simulink model "para_id_0_mod_corriente"  (R2018a)
settings: Solver=VariableStepAuto  StartTime=0.0  StopTime=10.0  RelTol=1e-3
values from neighbouring files (symbols this model uses):
  Beq = bm+(bl)/r^2    (= 1.5e-05)    [c4ModeloCompleto_var.m]
  Cts = .818    (= 0.818)    [c4ModeloCompleto.m]    (also in c4ModeloCompleto_var.m)
  Jeq = Jm+(Jl/r^2)    (= 5.65099476805e-06)    [c4ModeloCompleto_var.m]
  Ld = 6.6    [c4ModeloCompleto.m]    (also in c4ModeloCompleto_var.m = 0.0066)
  Lq = 5.8    [c4ModeloCompleto.m]    (also in c4ModeloCompleto_var.m = 0.0058)
  Pp = 3    [c4ModeloCompleto.m]    (also in c4ModeloCompleto_var.m)
  r = 314.3008    [c4ModeloCompleto.m]    (also in c4ModeloCompleto_var.m)
  Rs = 1.02    [c4ModeloCompleto_var.m]
  Rts_amb = 146.7    [c4ModeloCompleto.m]    (also in c4ModeloCompleto_var.m)
undefined symbols (not defined in the file or in its folder): L0
settings Model: Creator=agustin  LastModifiedBy=emanuel
settings CodeAppCC: StateflowObjectComments=on

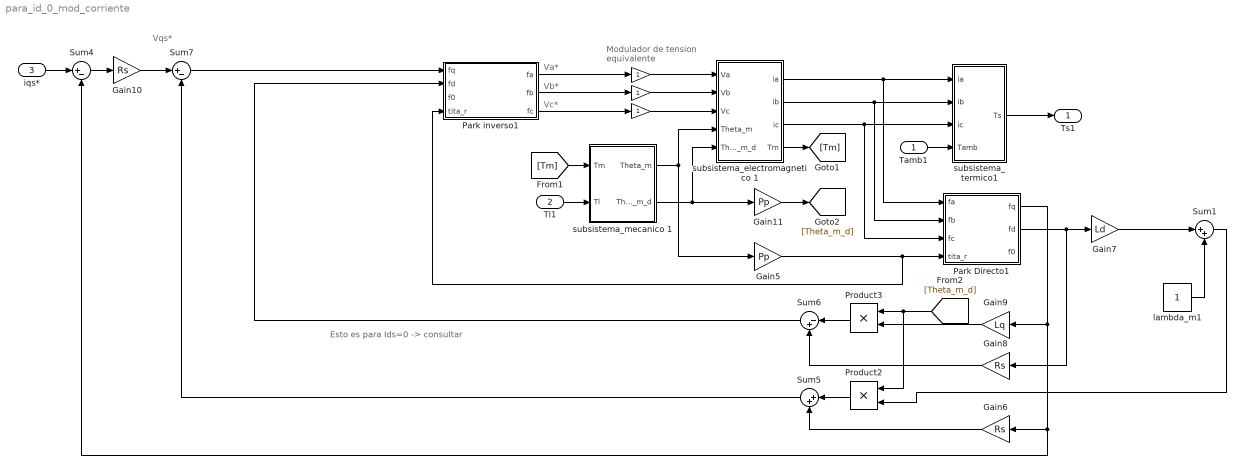
== system para_id_0_mod_corriente ==
  note: Vqs*
  note: Modulador de tension
      | equivalente
  note: Vc*
  note: Vb*
  note: Va*
  note: Esto es para Ids=0 -> consultar
  Tamb1 : Inport
  Tl1 : Inport  Port=2
  iqs* : Inport  Port=3
  " " : Gain
  " " : Gain
  " " : Gain
  Gain10 : Gain  Gain=Rs
  Gain11 : Gain  Gain=Pp
  Gain5 : Gain  Gain=Pp
  Gain6 : Gain  Gain=Rs
  Gain7 : Gain  Gain=Ld
  Gain8 : Gain  Gain=Rs
  Gain9 : Gain  Gain=Lq
  Park Directo1 : MATLAB Function  TreatAsAtomicUnit=on
  Park inverso1 : MATLAB Function  TreatAsAtomicUnit=on
  Product2 : Product
  Product3 : Product
  Sum1 : Sum  Inputs=|++
  Sum4 : Sum  Inputs=|+-
  Sum5 : Sum  Inputs=|++
  Sum6 : Sum  Inputs=|-+
  Sum7 : Sum  Inputs=|+-
  lambda_m1 : Constant
  subsistema_electromagnetico 1 : Subsystem
  subsistema_mecanico 1 : Subsystem
  subsistema_termico1 : Subsystem
  Ts1 : Outport
  wires:
  subsistema_mecanico 1/2("Theta_m_d ") -> Gain11/1, subsistema_electromagnetico 1/5(Theta_m_d)
  subsistema_termico1/1(Ts) -> Ts1/1
  Tamb1/1 -> subsistema_termico1/4(Tamb)
  subsistema_mecanico 1/1("Theta_m ") -> Gain5/1, subsistema_electromagnetico 1/4(Theta_m)
  Park inverso1/1(fa) -> " "/1
  Park inverso1/2(fb) -> " "/1
  Park inverso1/3(fc) -> " "/1
  subsistema_electromagnetico 1/1(ia) -> subsistema_termico1/1(ia), Park Directo1/1(fa)
  subsistema_electromagnetico 1/2(ib) -> Park Directo1/2(fb), subsistema_termico1/2(ib)
  subsistema_electromagnetico 1/3(ic) -> Park Directo1/3(fc), subsistema_termico1/3("ic ")
  Gain5/1 -> Park inverso1/4(tita_r), Park Directo1/4(tita_r)
  [Tm] -> subsistema_mecanico 1/1(Tm)
  subsistema_electromagnetico 1/4(Tm) -> [Tm]
  Tl1/1 -> subsistema_mecanico 1/2(Tl)
  Park Directo1/1(fq) -> Gain9/1, Sum4/2, Gain6/1
  Park Directo1/2(fd) -> Gain8/1, Gain7/1
  Gain7/1 -> Sum1/1
  lambda_m1/1 -> Sum1/2
  Sum1/1 -> Product2/2
  Gain6/1 -> Sum5/2
  Product2/1 -> Sum5/1
  Sum5/1 -> Sum7/2
  Gain8/1 -> Sum6/2
  Gain9/1 -> Product3/2
  Product3/1 -> Sum6/1
  Sum6/1 -> Park inverso1/2(fd)
  " "/1 -> subsistema_electromagnetico 1/1(Va)
  " "/1 -> subsistema_electromagnetico 1/3(Vc)
  " "/1 -> subsistema_electromagnetico 1/2(Vb)
  iqs*/1 -> Sum4/1
  Sum4/1 -> Gain10/1
  Gain10/1 -> Sum7/1
  [Theta_m_d] -> Product2/1, Product3/1
  Gain11/1 -> [Theta_m_d]
  Sum7/1 -> Park inverso1/1(fq)

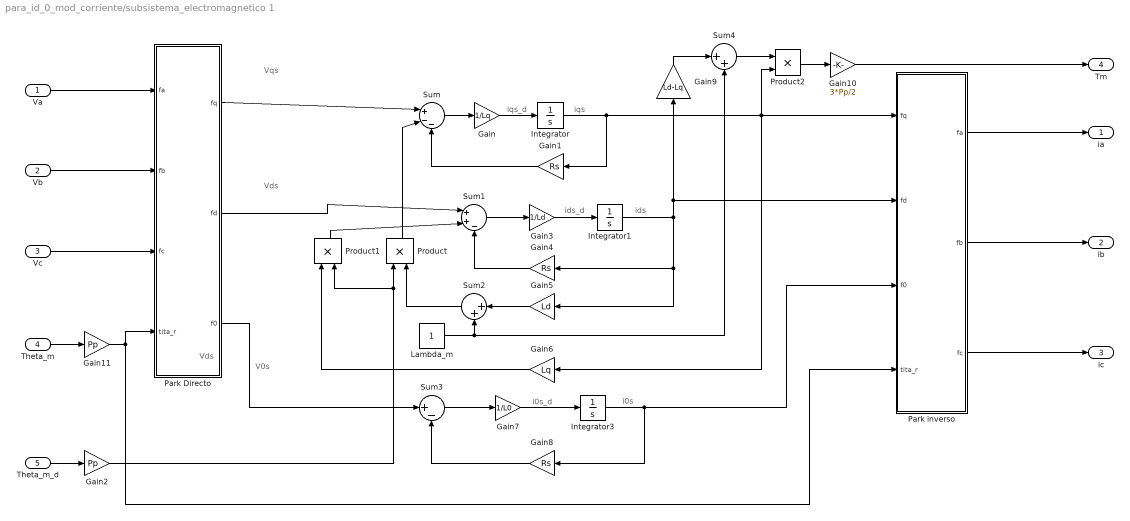
== system para_id_0_mod_corriente/subsistema_electromagnetico 1 ==
  note: Vds
  note: Vqs
  note: V0s
  note: Vds
  note: i0s
  note: i0s_d
  note: ids_d
  note: ids
  note: iqs
  note: iqs_d
  Va : Inport
  Vb : Inport  Port=2
  Vc : Inport  Port=3
  Theta_m : Inport  Port=4
  Theta_m_d : Inport  Port=5
  Gain : Gain  Gain=1/Lq
  Gain1 : Gain  Gain=Rs
  Gain10 : Gain  Gain=3*Pp/2
  Gain11 : Gain  Gain=Pp
  Gain2 : Gain  Gain=Pp
  Gain3 : Gain  Gain=1/Ld
  Gain4 : Gain  Gain=Rs
  Gain5 : Gain  Gain=Ld
  Gain6 : Gain  Gain=Lq
  Gain7 : Gain  Gain=1/L0
  Gain8 : Gain  Gain=Rs
  Gain9 : Gain  Gain=Ld-Lq
  Integrator : Integrator
  Integrator1 : Integrator
  Integrator3 : Integrator
  "Lambda_m " : Constant
  Park Directo : MATLAB Function  TreatAsAtomicUnit=on
  Park inverso : MATLAB Function  TreatAsAtomicUnit=on
  Product : Product
  Product1 : Product
  Product2 : Product
  Sum : Sum  Inputs=|+--
  Sum1 : Sum  Inputs=|++-
  Sum2 : Sum  Inputs=|++
  Sum3 : Sum  Inputs=|+-
  Sum4 : Sum  Inputs=|++
  ia : Outport
  ib : Outport  Port=2
  ic : Outport  Port=3
  Tm : Outport  Port=4
  wires:
  Product/1 -> Sum/2
  Theta_m_d/1 -> Gain2/1
  Product1/1 -> Sum1/2
  Gain2/1 -> Product1/2, Product/1
  Park Directo/3(f0) -> Sum3/1
  Integrator/1 -> Product2/2, Park inverso/1(fq), Gain6/1, Gain1/1
  Gain8/1 -> Sum3/2
  Sum2/1 -> Product/2
  Sum3/1 -> Gain7/1
  Park Directo/1(fq) -> Sum/1
  Sum/1 -> Gain/1
  Gain3/1 -> Integrator1/1
  Park Directo/2(fd) -> Sum1/1
  Gain4/1 -> Sum1/3
  Integrator1/1 -> Gain9/1, Park inverso/2(fd), Gain5/1, Gain4/1
  Sum1/1 -> Gain3/1
  Gain5/1 -> Sum2/1
  Gain/1 -> Integrator/1
  Gain6/1 -> Product1/1
  Gain1/1 -> Sum/3
  "Lambda_m "/1 -> Sum2/2, Sum4/2
  Gain7/1 -> Integrator3/1
  Integrator3/1 -> Park inverso/3(f0), Gain8/1
  Gain9/1 -> Sum4/1
  Sum4/1 -> Product2/1
  Product2/1 -> Gain10/1
  Gain10/1 -> Tm/1
  Vb/1 -> Park Directo/2(fb)
  Va/1 -> Park Directo/1(fa)
  Vc/1 -> Park Directo/3(fc)
  Theta_m/1 -> Gain11/1
  Gain11/1 -> Park inverso/4(tita_r), Park Directo/4(tita_r)
  Park inverso/1(fa) -> ia/1
  Park inverso/2(fb) -> ib/1
  Park inverso/3(fc) -> ic/1

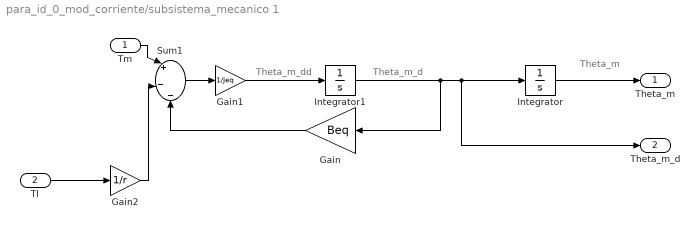
== system para_id_0_mod_corriente/subsistema_mecanico 1 ==
  note: Theta_m_dd
  note: Theta_m_d
  note: Theta_m
  Tm : Inport
  Tl : Inport  Port=2
  Gain : Gain  Gain=Beq
  Gain1 : Gain  Gain=1/Jeq
  Gain2 : Gain  Gain=1/r
  Integrator : Integrator
  Integrator1 : Integrator
  Sum1 : Sum  Inputs=|+|-|-
  "Theta_m " : Outport
  "Theta_m_d " : Outport  Port=2
  wires:
  Gain1/1 -> Integrator1/1
  Integrator1/1 -> Gain/1, "Theta_m_d "/1, Integrator/1
  Integrator/1 -> "Theta_m "/1
  Sum1/1 -> Gain1/1
  Tm/1 -> Sum1/1
  Gain/1 -> Sum1/3
  Tl/1 -> Gain2/1
  Gain2/1 -> Sum1/2

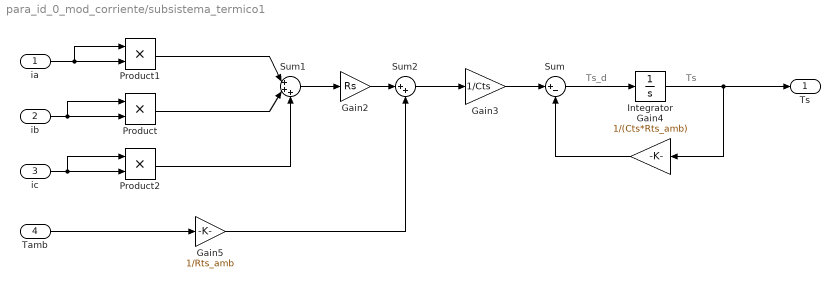
== system para_id_0_mod_corriente/subsistema_termico1 ==
  note: Ts
  note: Ts_d
  ia : Inport
  ib : Inport  Port=2
  "ic " : Inport  Port=3
  Tamb : Inport  Port=4
  Gain2 : Gain  Gain=Rs
  Gain3 : Gain  Gain=1/Cts
  Gain4 : Gain  Gain=1/(Cts*Rts_amb)
  Gain5 : Gain  Gain=1/Rts_amb
  Integrator : Integrator
  Product : Product
  Product1 : Product
  Product2 : Product
  Sum : Sum  Inputs=|+-
  Sum1 : Sum  Inputs=|+++
  Sum2 : Sum  Inputs=|++
  Ts : Outport
  wires:
  Gain4/1 -> Sum/2
  Sum1/1 -> Gain2/1
  Product2/1 -> Sum1/3
  Product/1 -> Sum1/2
  Integrator/1 -> Gain4/1, Ts/1
  ib/1 -> Product/2, Product/1
  "ic "/1 -> Product2/2, Product2/1
  Sum/1 -> Integrator/1
  Gain3/1 -> Sum/1
  Sum2/1 -> Gain3/1
  Product1/1 -> Sum1/1
  Gain5/1 -> Sum2/2
  Gain2/1 -> Sum2/1
  ia/1 -> Product1/2, Product1/1
  Tamb/1 -> Gain5/1

== matlab function para_id_0_mod_corriente/Park Directo1 ==
  data: fa input; fq output; fb input; fc input; tita_r input; fd output; f0 output
function [fq,fd,f0]     = t_park(fa,fb,fc,tita_r)

park_MATRIZ = [cos(tita_r) cos(tita_r-2*pi/3) cos(tita_r+2*pi/3); 
               sin(tita_r) sin(tita_r-2*pi/3) sin(tita_r+2*pi/3);
                  0.5           0.5            0.5];
                 
park_dir = (2/3) * park_MATRIZ * [fa;fb;fc];
fq = park_dir(1);
fd = park_dir(2);
f0 = park_dir(3);
end

== matlab function para_id_0_mod_corriente/Park inverso1 ==
  data: fq input; fd input; f0 input; tita_r input; fa output; fb output; fc output
function [fa, fb, fc] = t_park_inv(fq, fd , f0, tita_r)


park_MATRIZ = [cos(tita_r)        sin(tita_r)        1; 
               cos(tita_r-2*pi/3) sin(tita_r-2*pi/3) 1;
               cos(tita_r+2*pi/3) sin(tita_r+2*pi/3) 1];
                 
park_inv = park_MATRIZ * [fq;fd;f0];
fa = park_inv(1);
fb = park_inv(2);
fc = park_inv(3);
end

== matlab function para_id_0_mod_corriente/subsistema_electromagnetico 1/Park Directo ==
  data: fa input; fq output; fb input; fc input; tita_r input; fd output; f0 output
function [fq,fd,f0]     = t_park(fa,fb,fc,tita_r)

park_MATRIZ = [cos(tita_r) cos(tita_r-2*pi/3) cos(tita_r+2*pi/3); 
               sin(tita_r) sin(tita_r-2*pi/3) sin(tita_r+2*pi/3);
                  0.5           0.5            0.5];
                 
park_dir = (2/3) * park_MATRIZ * [fa;fb;fc];
fq = park_dir(1);
fd = park_dir(2);
f0 = park_dir(3);
end

== matlab function para_id_0_mod_corriente/subsistema_electromagnetico 1/Park inverso ==
  data: fq input; fd input; f0 input; tita_r input; fa output; fb output; fc output
function [fa, fb, fc] = t_park_inv(fq, fd , f0, tita_r)


park_MATRIZ = [cos(tita_r)        sin(tita_r)        1; 
               cos(tita_r-2*pi/3) sin(tita_r-2*pi/3) 1;
               cos(tita_r+2*pi/3) sin(tita_r+2*pi/3) 1];
                 
park_inv = park_MATRIZ * [fq;fd;f0];
fa = park_inv(1);
fb = park_inv(2);
fc = park_inv(3);
end
